simulink model "RC_ckt"  (R2020a)
settings: Solver=VariableStepAuto  StartTime=0.0  StopTime=10.0  RelTol=1e-3
model workspace (MAT data in the model file):
  C = 0.001
  R = 10
settings Model: Creator=Shubham  LastModifiedBy=Shubham

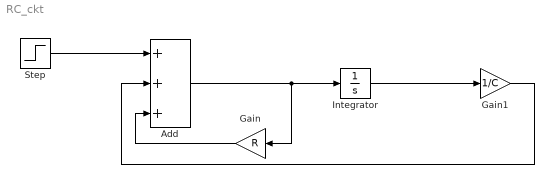
== system RC_ckt ==
  Add : Sum  Inputs=+++
  Gain : Gain  Gain=R
  Gain1 : Gain  Gain=1/C
  Integrator : Integrator
  Step : Step  SampleTime=0
  wires:
  Step/1 -> Add/1
  Add/1 -> Gain/1, Integrator/1
  Integrator/1 -> Gain1/1
  Gain1/1 -> Add/2
  Gain/1 -> Add/3
